simulink model "vehicle_hostmodel_2022b"  (R2022b)
settings: Solver=VariableStepAuto  StartTime=0.0  StopTime=inf  RelTol=1e-3
model workspace (MAT data in the model file):
  firstWarning = 1
  originalScenarioChecksum = '114339432DE22364D47BB28FC96DC10C'
undefined symbols (not defined in the file or in its folder): Acceleration, ActorID, AngularVelocity, curvature, DefaultGear, DEND_B, DEND_S, DEND_T, direction, DiscIntNeverNeededParam, driving, gradbp, L, LF, LR, matlabshared, MAX_BRAKE, MAX_STEER, MAX_TORQUE, MCAR, MIN_BRAKE, MIN_STEER, MIN_TORQUE, NUMD_B, NUMD_S, NUMD_T, Pitch, Position, psi_o, R, Roll, RRdamp, SceneInfo, session, sigbuilder_block, STEER_RATIO, stopSign_ID, Tdead, thetaRefs, TL_ID, TrackWidth, Ts, ts, Vdead, Velocity, WB, X_o, xRef2s, Y_o, Yaw, yRef2, yRef2s
libraries: drivingscenarioandsensors x8, slrealtimeutilitieslib x7, slrealtimeiplib x7, simulink x6, drivingvehiclecontroller x2, slpidlib x2, trackingutilitieslib x2, simulink_extras x2, robotalgslib x1, eeGeneralControl x1, mpcadaslib x1, drivinglib x1
(part 1 of 4)
settings Model: Creator=akshran  LastModifiedBy=giridhar.9
settings DataIOCC: SignalLogging=off
settings DebuggingCC: UnconnectedInputMsg=warning  UnconnectedOutputMsg=warning  UnconnectedLineMsg=warning
settings ModelReferenceCC: EnableRefExpFcnMdlSchedulingChecks=on
settings RTWCC: DLArmComputeVersion=19.05

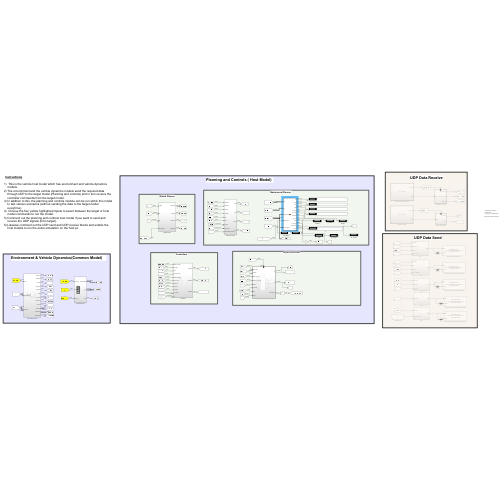
[thumbnail: Simulink's stored preview of the top-level diagram]
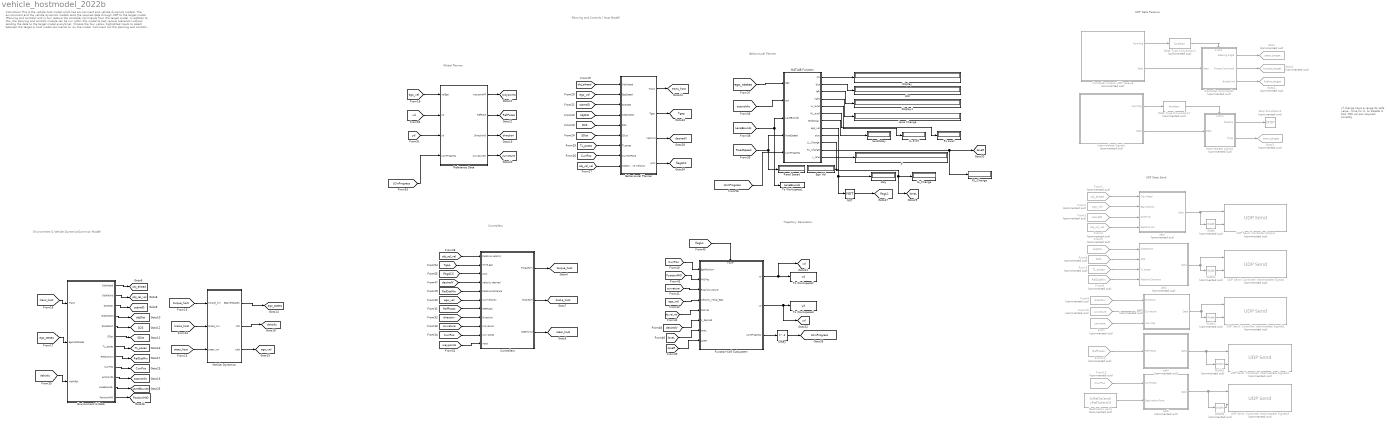
== system vehicle_hostmodel_2022b ==
  note: Global Planner
  note: xf change have a range
      | ttc safe value
      | - time for lc, to disable lc blok
      |
      | MIO vel pos required correctly
  note: Trajectory Generation
  note: Behavioural Planner
  note: Instructions
      |
      | This is the vehicle host model which has environment and vehicle dynamics models.
      | The environment and the vehicle dynamics models send the required data through UDP to the target model (Planning and controls) and in turn receive the controller commands from the target model.
      | In addition to this, the planning and controls module can be run within this model to test various scenarios (without sending the data to the target model everytime).
      | Choose the four yellow highlighted inputs to select between the target or host model commands to run the model.
      | Comment out the planning and controls host model if you want to send and receive the UDP signals (from target).
      | Likewise comment out the UDP send and UDP receive blocks and enable the host models to run the entire simulation on the host pc.
  note: Environment & Vehicle Dynamics(Common Model)
  note: UDP Data Receive
  note: UDP Data Send
  note: Planning and Controls ( Host Model)
  note: Controllers
  Behavioural Planner : Subsystem
  Controller commands : Subsystem  Commented=on
  Controller output- UDP receive : Subsystem  Commented=on
  Controllers : Subsystem
  Data Type Conversion1 : DataTypeConversion  Commented=on  OutDataTypeStr=boolean  SaturateOnIntegerOverflow=off  RndMeth=Floor
  Data Type Conversion2 : DataTypeConversion  Commented=on  OutDataTypeStr=boolean  SaturateOnIntegerOverflow=off  RndMeth=Floor
  Delay : Delay  DelayLength=1
  Destination point : Constant  Commented=on  Value=[xRef2s(end) yRef2s(end)]
  Display : Display
  Display1 : Display
  Ego Vel : Display
  Environment & Data : Subsystem
  From : From  Commented=on  GotoTag=yawrate  TagVisibility=global
  From1 : From  Commented=on  GotoTag=obj_ahead  TagVisibility=global
  From10 : From  Commented=on  GotoTag=curvature  TagVisibility=global
  From11 : From  Commented=on  GotoTag=RefPoses  TagVisibility=global
  From12 : From  Commented=on  GotoTag=CurrPos  TagVisibility=global
  From2 : From  Commented=on  GotoTag=ego_vel  TagVisibility=global
  From3 : From  Commented=on  GotoTag=sceneID  TagVisibility=global
  From4 : From  Commented=on  GotoTag=obj_rel_vel  TagVisibility=global
  From5 : From  Commented=on  GotoTag=objDist  TagVisibility=global
  From6 : From  Commented=on  GotoTag=D2S  TagVisibility=global
  From7 : From  Commented=on  GotoTag=TL_poses  TagVisibility=global
  From8 : From  Commented=on  GotoTag=RelDistMin  TagVisibility=global
  From9 : From  Commented=on  GotoTag=direction  TagVisibility=global
  Function-Call Subsystem : Subsystem  TreatAsAtomicUnit=on
  Goto : Goto  Commented=on  GotoTag=steer_target  TagVisibility=global
  Goto1 : Goto  Commented=on  GotoTag=torque_target  TagVisibility=global
  Goto2 : Goto  Commented=on  GotoTag=brake_target  TagVisibility=global
  Goto3 : Goto  Commented=on  GotoTag=trans_target  TagVisibility=global
  Intermediate Signals : Subsystem  Commented=on
  Intermediate signals : Subsystem  Commented=on
  LL avail : Display
  LL_Change : Display
  "Lane Change " : Display
  MATLAB Function : MATLAB Function  TreatAsAtomicUnit=on
  NOT : Logic  Operator=NOT  IconShape=distinctive  AllPortsSameDT=off  OutDataTypeStr=boolean
  RL avail : Display
  RL_Change : Display
  Reference Data : Subsystem  VariantControl=Stanley
  Road Speed : Display
  Stop Simulation1 : Stop  Commented=on
  To Workspace1 : ToWorkspace  VariableName=LaneBounds  SaveFormat=Timeseries  SampleTime=-1
  To Workspace2 : ToWorkspace  VariableName=xd  SampleTime=-1
      settings: Save2DSignal=2-D array (concatenate along first dimension)
  To Workspace3 : ToWorkspace  VariableName=yd  SampleTime=-1
      settings: Save2DSignal=2-D array (concatenate along first dimension)
  UDP Send: Controller Intermediate Signals : slrealtimeiplib/UDP Send  Commented=on  useHostTargetConn=on  toAddress=192.168.7.2  toPort=8002  sampleTime=0.1  enableMessage=off  ipAddress=192.168.7.2  localPort=-1
  UDP Send: Controller Intermediate Signals1 : slrealtimeiplib/UDP Send  Commented=on  useHostTargetConn=on  toAddress=192.168.7.2  toPort=8003  sampleTime=0.1  enableMessage=off  ipAddress=192.168.7.2  localPort=-1
  UDP Send: Controller Intermediate Signals2 : slrealtimeiplib/UDP Send  Commented=on  useHostTargetConn=on  toAddress=192.168.7.2  toPort=8004  sampleTime=0.1  enableMessage=off  ipAddress=192.168.7.2  localPort=-1
  UDP Send: Controller Intermediate Signals3 : slrealtimeiplib/UDP Send  Commented=on  useHostTargetConn=on  toAddress=192.168.7.2  toPort=8005  sampleTime=0.1  enableMessage=off  ipAddress=192.168.7.2  localPort=-1
  UDP Send: Controller Output : slrealtimeiplib/UDP Send  Commented=on  useHostTargetConn=on  toAddress=192.168.7.2  toPort=8001  sampleTime=0.1  enableMessage=off  ipAddress=192.168.7.2  localPort=-1
  Vehicle Dynamics : Subsystem
  Width{,1..4} (5 alike) : Width  Commented=on
  d : Display
  dist : Display
  set1 : Subsystem  Commented=on
  set2 : Subsystem  Commented=on
  set3 : Subsystem  Commented=on
  set4 : Subsystem  Commented=on
  set5 : Subsystem  Commented=on
  stay : Display
  tend2stay : Display
  tag scope: CurrPos=global, D2S=global, LCinProgress=global, LaneBounds=global, PositionMIO=global, RefPoses=global, RelDistMin=global, SDist=global, TL_poses=global, Tgap=global, VehInfo=global, actorsInfo=global, brake_host=global, curvature=global, desiredV=global, direction=global, ego_states=global, ego_vel=global, flagACC=global, flagLC=global, laneL=global, laneR=global, objDist=global, obj_ahead=global, obj_rel_vel=global, sceneID=global, steer_host=global, torque_host=global, trans_host=global, waypoints=global, xd=global, yd=global
  wires:
  Behavioural Planner/3(VelCmd) -> [desiredV]
  Width/1 -> UDP Send: Controller Output/2
  Width1/1 -> UDP Send: Controller Intermediate Signals/2
  set1/1(Data) -> Width/1, UDP Send: Controller Output/1
  set2/1(Data) -> UDP Send: Controller Intermediate Signals/1, Width1/1
  set3/1(Data) -> UDP Send: Controller Intermediate Signals1/1, Width2/1
  Width2/1 -> UDP Send: Controller Intermediate Signals1/2
  Width3/1 -> UDP Send: Controller Intermediate Signals2/2
  set4/1(Data) -> Width3/1, UDP Send: Controller Intermediate Signals2/1
  set5/1(Data) -> Width4/1, UDP Send: Controller Intermediate Signals3/1
  Width4/1 -> UDP Send: Controller Intermediate Signals3/2
  From/1 -> set3/3(yaw rate)
  Controller output- UDP receive/2(Data) -> Controller commands/1(Data)
  Controller output- UDP receive/1(NumMsg) -> Data Type Conversion2/1
  Data Type Conversion2/1 -> Controller commands/Enable
  Data Type Conversion1/1 -> Intermediate signals/Enable
  Intermediate Signals/1(NumMsg) -> Data Type Conversion1/1
  Intermediate Signals/2(Data) -> Intermediate signals/1(Data)
  Intermediate signals/1(StopSim) -> Stop Simulation1/1
  Destination point/1 -> set5/2(Destination Point)
  Controller commands/1(Steering Angle) -> Goto/1
  Controller commands/2(Torque Command) -> Goto1/1
  Controller commands/3(BrakeCmd) -> Goto2/1
  Intermediate signals/2(Trans) -> Goto3/1
  Controllers/1(TorgueCm) -> [torque_host]
  Controllers/2(BrakeCm) -> [brake_host]
  Controllers/3(SteerCmd) -> [steer_host]
  Environment & Data/1(ObjAhead) -> [obj_ahead]
  Environment & Data/2(ObjRelVel) -> [obj_rel_vel]
  Environment & Data/3(SceneID) -> [sceneID]
  Environment & Data/4(ObjectDist) -> [objDist]
  Environment & Data/6(SDist) -> [SDist]
  Environment & Data/5(SceneDist) -> [D2S]
  Environment & Data/7(TL_poses) -> [TL_poses]
  Vehicle Dynamics/1(EgoVehStates) -> [ego_states]
  Vehicle Dynamics/3(xdot) -> [ego_vel]
  Environment & Data/8(RelDistmin) -> [RelDistMin]
  Vehicle Dynamics/2(Info) -> [VehInfo]
  Behavioural Planner/1(Trans) -> [trans_host]
  From1/1 -> set1/1(Obj Ahead)
  From2/1 -> set1/2(Ego Velocity)
  From3/1 -> set1/3(Scene ID)
  From4/1 -> set1/4(Relative Vel)
  From5/1 -> set2/1(ObjectDist)
  From6/1 -> set2/2(D2S)
  From7/1 -> set2/3(TL poses)
  From8/1 -> set2/4(Relative Distance)
  From9/1 -> set3/1(Direction)
  From10/1 -> set3/2(Curvature)
  From11/1 -> set4/1(Ref Poses)
  From12/1 -> set5/1(CurrPoses)
  [torque_host] -> Vehicle Dynamics/1(torque_cm)
  [brake_host] -> Vehicle Dynamics/2(brake_cm)
  [steer_host] -> Vehicle Dynamics/3(steer_cm)
  [trans_host] -> Environment & Data/1(Trans)
  [ego_states] -> Environment & Data/2(EgoVehStates)
  [obj_ahead] -> Behavioural Planner/1(ObjAhead)
  [ego_vel] -> Behavioural Planner/2(EgoSpeed)
  [sceneID] -> Behavioural Planner/3(SceneID)
  [objDist] -> Behavioural Planner/4(ObjectDist)
  [D2S] -> Behavioural Planner/5(D2S)
  [SDist] -> Behavioural Planner/6(SDist)
  [TL_poses] -> Behavioural Planner/7(TLposes)
  [CurrPos] -> Behavioural Planner/8(CurrentPose)
  [obj_rel_vel] -> Behavioural Planner/9(Object Relative Velocity)
  [obj_rel_vel] -> Controllers/1(Relative velocity)
  [RelDistMin] -> Controllers/5(Relative distance)
  [ego_vel] -> Controllers/6(CurrVelocity)
  [RefPoses] -> Controllers/7(RefPoses)
  [direction] -> Controllers/8(Direction)
  [curvature] -> Controllers/9(Curvature)
  [CurrPos] -> Controllers/10(curr poses)
  [VehInfo] -> Environment & Data/3(VehFdbk)
  Environment & Data/9(CurrPos) -> [CurrPos]
  Environment & Data/10(actorsinfo) -> [actorsInfo]
  [ego_states] -> MATLAB Function/1(ego)
  [actorsInfo] -> MATLAB Function/2(act)
  MATLAB Function/1(ttc) -> Display/1
  Environment & Data/11(LaneBounds) -> [LaneBounds]
  [LaneBounds] -> MATLAB Function/3(LaneBounds), To Workspace1/1
  MATLAB Function/3(left) -> Display1/1
  MATLAB Function/4(right) -> "Lane Change "/1
  MATLAB Function/2(dist) -> dist/1
  [RoadSpeed] -> Road Speed/1, MATLAB Function/4(RoadSpeed)
  MATLAB Function/8(ego_vel) -> Ego Vel/1
  MATLAB Function/6(RL_avail) -> RL avail/1
  MATLAB Function/5(LL_avail) -> LL avail/1
  MATLAB Function/7(tend2stay) -> tend2stay/1
  MATLAB Function/9(stay) -> NOT/1, stay/1
  MATLAB Function/10(LL_Change) -> LL_Change/1, [laneL]
  MATLAB Function/11(RL_Change) -> RL_Change/1, [laneR]
  MATLAB Function/12(y_lane) -> d/1
  [CurrPos] -> Function-Call Subsystem/1(EgoPosition)
  [curvature] -> Function-Call Subsystem/3(Road Curvature)
  [ego_vel] -> Function-Call Subsystem/4(Velocity_Initial_Ego)
  Environment & Data/12(PositionMIO) -> [PositionMIO]
  [PositionMIO] -> Function-Call Subsystem/2(MIOPos)
  [obj_rel_vel] -> Function-Call Subsystem/5(MIOVel)
  NOT/1 -> [flagLC]
  Function-Call Subsystem/1(xd) -> [xd], To Workspace2/1
  Function-Call Subsystem/2(yd) -> [yd], To Workspace3/1
  [desiredV] -> Function-Call Subsystem/6(V_desired)
  [desiredV] -> Controllers/4(velocity desired)
  [laneR] -> Function-Call Subsystem/8(laneR)
  [laneL] -> Function-Call Subsystem/7(laneL)
  [flagLC] -> Function-Call Subsystem/Trigger
  [ego_vel] -> Reference Data/1(velEgo)
  Reference Data/1(waypointPP) -> [waypoints]
  Reference Data/2(RefPose) -> [RefPoses]
  Reference Data/3(DirectionO) -> [direction]
  [xd] -> Reference Data/2(xd)
  [yd] -> Reference Data/3(yd)
  [waypoints] -> Controllers/11(Input)
  Reference Data/4(CurvatureO) -> [curvature]
  [LCinProgress] -> Reference Data/4(LCinProgress)
  Behavioural Planner/2(Tgap) -> [Tgap]
  Behavioural Planner/4(ACC) -> [flagACC]
  [Tgap] -> Controllers/2(Time gap)
  [flagACC] -> Controllers/3(ACC)
  Function-Call Subsystem/3(LCinProgress) -> Delay/1
  Delay/1 -> [LCinProgress]
  [LCinProgress] -> MATLAB Function/5(LCinProgress)

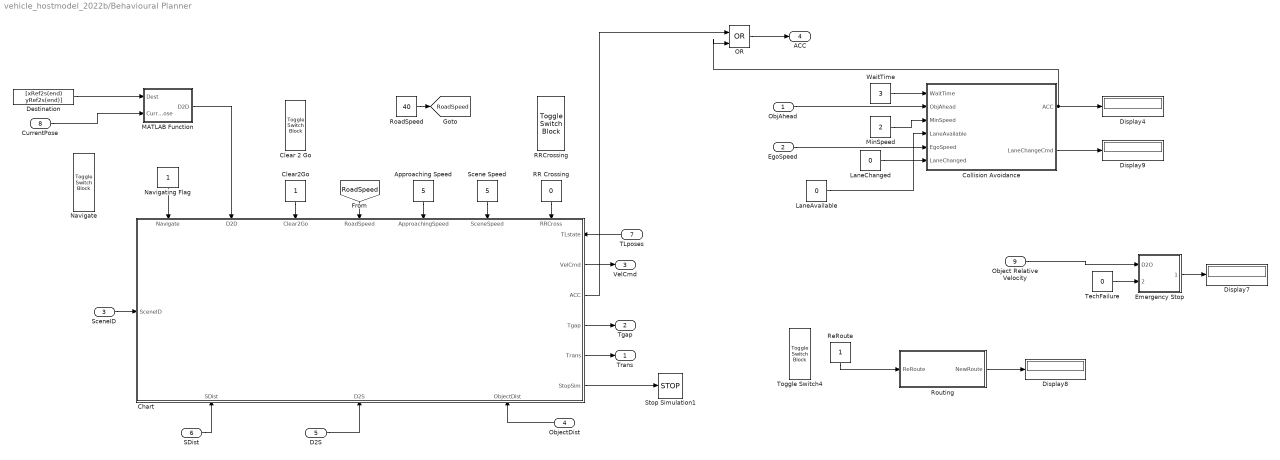
== system vehicle_hostmodel_2022b/Behavioural Planner ==
  ObjAhead : Inport
  EgoSpeed : Inport  Port=2
  SceneID : Inport  Port=3
  ObjectDist : Inport  Port=4
  D2S : Inport  Port=5
  SDist : Inport  Port=6
  TLposes : Inport  Port=7
  CurrentPose : Inport  Port=8
  Object Relative Velocity : Inport  Port=9
  Approaching Speed : Constant  Value=5
  Chart : Stateflow chart  TreatAsAtomicUnit=on
      settings: PortSchema="{\"entries\":[{\"content\":{\"sides\":[{\"content\":{\"connectorIds\":[\"In12\"]},\"type\":\"ConnectorPlacement.EquallySpacedRectSide\",\"uuid\":\"81aca70f-0947-49fb-b60a-be241e44193b\"},{\"content\":{\"connectorIds\":[\"In1\",\"Out1\",\"Out2\",\"Out3\",\"Out4\",\"Out5\"],\"side\":\"RIGHT\"},\"type\":\"ConnectorPlacement.EquallySpacedRectSide\",\"uuid\":\"e7b9645e-3711-4964-ac9b-0199dd335e99\"},{\"content\":{\"connectorIds\":[\"In8\",\"In9\",\"In10\",\"In11\",\"In2\",\"In4\",\"In6\"],\"side\":\"TOP\"},\"type\":\"ConnectorPlacement.EquallySpacedRectSide\",\"uuid\":\"6876f024-944b-4540-9404-d68f37763657\"},{\"content\":{\"connectorIds\":[\"In5\",\"In7\",\"In3\"],\"side\":\"BOTTOM\"},\"type\":\"ConnectorPlacement.EquallySpacedRectSide\",\"uuid\":\"44acab73-cdde-4edf-95df-27422644ccab\"}]},\"type\":\"ConnectorPlacement.EquallySpacedConnector\",\"uuid\":\"d2c31c01-e447-43db-8d2b-8b98a0ca291a\"}],\"packageUris\":[\"http://schema.mathworks.com/mf0/Connector/R2020b\"],\"version\":\"1.0\"}"
  Clear 2 Go : ToggleSwitchBlock
      settings: Values={{'Off', 'On'}, [0 1]}
  Clear2Go : Constant
  Collision Avoidance : Stateflow chart  TreatAsAtomicUnit=on
  Destination : Constant  Value=[xRef2s(end) yRef2s(end)]
  Display{4,7..9} (4 alike) : Display
  Emergency Stop : Stateflow chart  TreatAsAtomicUnit=on
  LaneAvailable : Constant  Value=0
  LaneChanged : Constant  Value=0
  MATLAB Function : MATLAB Function  TreatAsAtomicUnit=on
  MinSpeed : Constant  Value=2
  Navigate : ToggleSwitchBlock
      settings: Values={{'Off', 'On'}, [0 1]}
  Navigating Flag : Constant
  OR : Logic  Operator=OR  IconShape=distinctive  AllPortsSameDT=off  OutDataTypeStr=fixdt(1,16)
  RR Crossing : Constant  Value=0
  RRCrossing : ToggleSwitchBlock
      settings: Values={{'Off', 'On'}, [0 1]}
  ReRoute : Constant
  RoadSpeed : Constant  Value=40
  Routing : Stateflow chart  TreatAsAtomicUnit=on
  Scene Speed : Constant  Value=5
  Stop Simulation1 : Stop
  TechFailure : Constant  Value=0
  Toggle Switch4 : ToggleSwitchBlock
      settings: Values={{'Off', 'On'}, [0 1]}
  WaitTime : Constant  Value=3
  Trans : Outport
  Tgap : Outport  Port=2
  VelCmd : Outport  Port=3
  ACC : Outport  Port=4
  tag scope: RoadSpeed=global
  wires:
  Clear2Go/1 -> Chart/10(Clear2Go)
  Routing/1(NewRoute) -> Display8/1
  ObjectDist/1 -> Chart/3(ObjectDist)
  WaitTime/1 -> Collision Avoidance/1(WaitTime)
  Navigating Flag/1 -> Chart/8(Navigate)
  Approaching Speed/1 -> Chart/2(ApproachingSpeed)
  Scene Speed/1 -> Chart/4(SceneSpeed)
  EgoSpeed/1 -> Collision Avoidance/5(EgoSpeed)
  ReRoute/1 -> Routing/1(ReRoute)
  Collision Avoidance/2(LaneChangeCmd) -> Display9/1
  LaneAvailable/1 -> Collision Avoidance/4(LaneAvailable)
  CurrentPose/1 -> MATLAB Function/2(CurrentPose)
  RR Crossing/1 -> Chart/6(RRCross)
  MinSpeed/1 -> Collision Avoidance/3(MinSpeed)
  LaneChanged/1 -> Collision Avoidance/6(LaneChanged)
  [RoadSpeed] -> Chart/11(RoadSpeed)
  ObjAhead/1 -> Collision Avoidance/2(ObjAhead)
  Destination/1 -> MATLAB Function/1(Dest)
  SceneID/1 -> Chart/12(SceneID)
  MATLAB Function/1(D2D) -> Chart/9(D2D)
  Chart/5(StopSim) -> Stop Simulation1/1
  Chart/4(Trans) -> Trans/1
  TLposes/1 -> Chart/1(TLstate)
  Chart/1(VelCmd) -> VelCmd/1
  SDist/1 -> Chart/5(SDist)
  D2S/1 -> Chart/7(D2S)
  Chart/3(Tgap) -> Tgap/1
  TechFailure/1 -> Emergency Stop/2(TechFailure)
  Emergency Stop/1(EStop) -> Display7/1
  Object Relative Velocity/1 -> Emergency Stop/1(D2O)
  Collision Avoidance/1(ACC) -> OR/2, Display4/1
  OR/1 -> ACC/1
  Chart/2(ACC) -> OR/1
  RoadSpeed/1 -> [RoadSpeed]

== system vehicle_hostmodel_2022b/Controller commands ==
  Data : Inport
  Enable : EnablePort
  "Byte Unpacking " : slrealtimeutilitieslib/Byte Unpacking  MaskUnpackedDataTypes={'double', 'double', 'double'}  MaskUnpackedDataSizes={[1], [1], [1]}  MaskAlignment=1
  Steering Angle : Outport
  Torque Command : Outport  Port=2
  BrakeCmd : Outport  Port=3
  wires:
  Data/1 -> "Byte Unpacking "/1
  "Byte Unpacking "/1 -> Steering Angle/1  "Steering angle"
  "Byte Unpacking "/2 -> Torque Command/1  "Longitudinal velocity"
  "Byte Unpacking "/3 -> BrakeCmd/1  "BrakeCmd"

== system vehicle_hostmodel_2022b/Controller output- UDP receive ==
  Compare To Constant : simulink/Logic and Bit Operations/Compare To Constant  relop===  const=24  OutDataTypeStr=boolean
  Constant : Constant
  Subtract : Sum  Inputs=+-
  UDP Receive2 : slrealtimeiplib/UDP Receive  useHostTargetConn=on  ipAddress=192.168.7.2  localPort=8016  rcvWidth=24  rcvFmAny=off  fmAddress=192.168.7.2  sampleTime=-1  enableMessage=off  maxPackets=1
  While Iterator : WhileIterator  WhileBlockType=do-while  ResetStates=reset  ShowIterationPort=on
  NumMsg : Outport
  Data : Outport  Port=2
  wires:
  Compare To Constant/1 -> While Iterator/1
  UDP Receive2/1 -> Data/1
  Constant/1 -> Subtract/2
  Subtract/1 -> NumMsg/1
  UDP Receive2/2 -> Compare To Constant/1
  While Iterator/1 -> Subtract/1

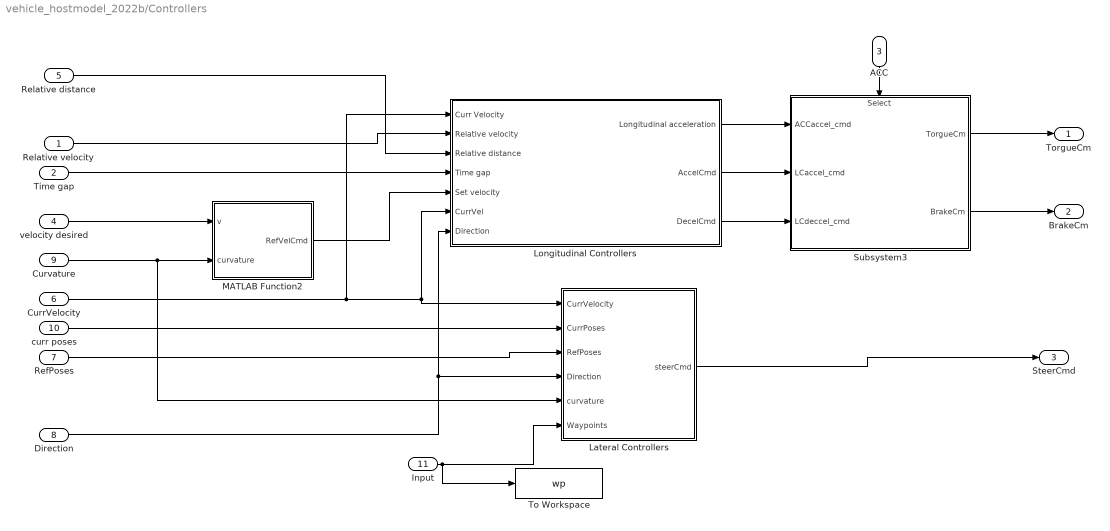
== system vehicle_hostmodel_2022b/Controllers ==
  Relative velocity : Inport
  Time gap : Inport  Port=2
  ACC : Inport  Port=3
  velocity desired : Inport  Port=4
  Relative distance : Inport  Port=5
  CurrVelocity : Inport  Port=6
  RefPoses : Inport  Port=7
  Direction : Inport  Port=8
  Curvature : Inport  Port=9
  curr poses : Inport  Port=10
  Input : Inport  Port=11
  Lateral Controllers : Subsystem
  Longitudinal Controllers : Subsystem
  MATLAB Function2 : MATLAB Function  TreatAsAtomicUnit=on
  Subsystem3 : Subsystem
      settings: PortSchema="{\"entries\":[{\"content\":{\"sides\":[{\"content\":{\"connectorIds\":[\"In1\",\"In2\",\"In3\"]},\"type\":\"ConnectorPlacement.EquallySpacedRectSide\",\"uuid\":\"a23b1a10-3bcb-40a0-900c-c9a3f160b173\"},{\"content\":{\"connectorIds\":[\"Out1\",\"Out2\"],\"side\":\"RIGHT\"},\"type\":\"ConnectorPlacement.EquallySpacedRectSide\",\"uuid\":\"88840b66-912f-4184-aeec-297642319416\"},{\"content\":{\"connectorIds\":[\"In4\"],\"side\":\"TOP\"},\"type\":\"ConnectorPlacement.EquallySpacedRectSide\",\"uuid\":\"37a03ca9-b065-473e-b290-3b07703c6005\"}]},\"type\":\"ConnectorPlacement.EquallySpacedConnector\",\"uuid\":\"5bfc7c71-8f7a-4cba-a168-7eeca22a2fcb\"}],\"packageUris\":[\"http://schema.mathworks.com/mf0/Connector/R2020b\"],\"version\":\"1.0\"}"
  To Workspace : ToWorkspace  VariableName=wp  SampleTime=-1
  TorgueCm : Outport
  BrakeCm : Outport  Port=2
  SteerCmd : Outport  Port=3
  wires:
  Longitudinal Controllers/1(Longitudinal acceleration) -> Subsystem3/1(ACCaccel_cmd)
  Curvature/1 -> MATLAB Function2/2(curvature), Lateral Controllers/5(curvature)
  Relative velocity/1 -> Longitudinal Controllers/2(Relative velocity)
  MATLAB Function2/1(RefVelCmd) -> Longitudinal Controllers/5(Set velocity)
  Direction/1 -> Longitudinal Controllers/7(Direction), Lateral Controllers/4(Direction)
  RefPoses/1 -> Lateral Controllers/3(RefPoses)
  velocity desired/1 -> MATLAB Function2/1(v)
  Longitudinal Controllers/2(AccelCmd) -> Subsystem3/2(LCaccel_cmd)
  Longitudinal Controllers/3(DecelCmd) -> Subsystem3/3(LCdeccel_cmd)
  CurrVelocity/1 -> Longitudinal Controllers/1(Curr Velocity), Longitudinal Controllers/6(CurrVel), Lateral Controllers/1(CurrVelocity)
  Time gap/1 -> Longitudinal Controllers/4(Time gap)
  Relative distance/1 -> Longitudinal Controllers/3(Relative distance)
  Lateral Controllers/1(steerCmd) -> SteerCmd/1
  ACC/1 -> Subsystem3/4(Select)
  curr poses/1 -> Lateral Controllers/2(CurrPoses)
  Subsystem3/1(TorgueCm) -> TorgueCm/1
  Subsystem3/2(BrakeCm) -> BrakeCm/1
  Input/1 -> To Workspace/1, Lateral Controllers/6(Waypoints)

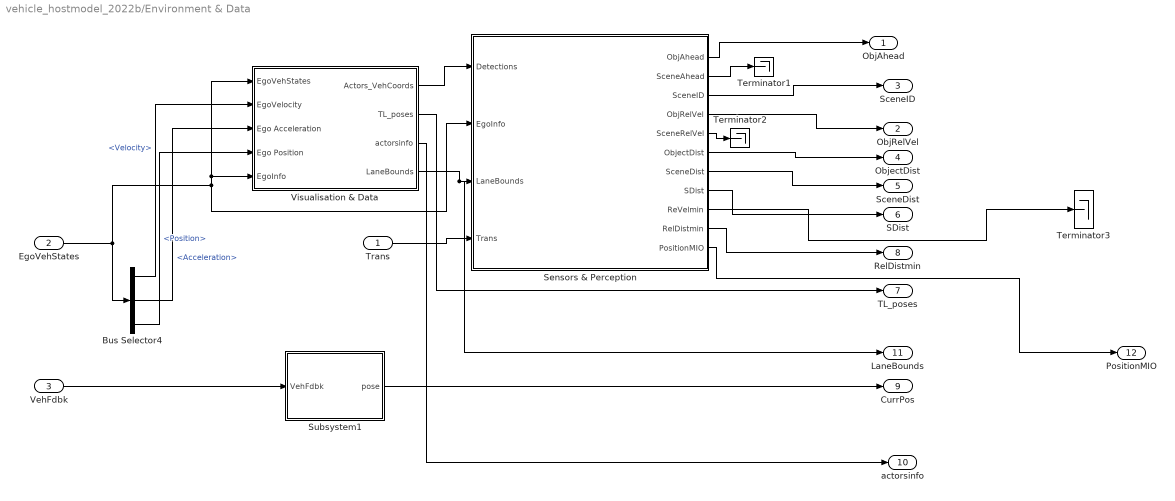
== system vehicle_hostmodel_2022b/Environment & Data ==
  Trans : Inport
  EgoVehStates : Inport  Port=2
  VehFdbk : Inport  Port=3
  Bus Selector4 : BusSelector  OutputSignals=Velocity,Acceleration,Position
  Sensors & Perception : Subsystem
  Subsystem1 : Subsystem
  Terminator1 : Terminator
  Terminator2 : Terminator
  Terminator3 : Terminator
  Visualisation & Data : Subsystem
  ObjAhead : Outport
  ObjRelVel : Outport  Port=2
  SceneID : Outport  Port=3
  ObjectDist : Outport  Port=4
  SceneDist : Outport  Port=5
  SDist : Outport  Port=6
  TL_poses : Outport  Port=7
  RelDistmin : Outport  Port=8
  CurrPos : Outport  Port=9
  actorsinfo : Outport  Port=10
  LaneBounds : Outport  Port=11
  PositionMIO : Outport  Port=12
  wires:
  Bus Selector4/3 -> Visualisation & Data/4(Ego Position)  "<Position>"
  Sensors & Perception/1(ObjAhead) -> ObjAhead/1
  Bus Selector4/1 -> Visualisation & Data/2(EgoVelocity)  "<Velocity>"
  Visualisation & Data/1(Actors_VehCoords) -> Sensors & Perception/1(Detections)
  Sensors & Perception/5(SceneRelVel) -> Terminator2/1
  Sensors & Perception/2(SceneAhead) -> Terminator1/1
  Sensors & Perception/6(ObjectDist) -> ObjectDist/1
  Bus Selector4/2 -> Visualisation & Data/3(Ego Acceleration)  "<Acceleration>"
  Sensors & Perception/9(ReVelmin) -> Terminator3/1
  EgoVehStates/1 -> Visualisation & Data/5(EgoInfo), Visualisation & Data/1(EgoVehStates), Sensors & Perception/2(EgoInfo), Bus Selector4/1
  Sensors & Perception/4(ObjRelVel) -> ObjRelVel/1
  Visualisation & Data/2(TL_poses) -> TL_poses/1
  Sensors & Perception/3(SceneID) -> SceneID/1
  Sensors & Perception/8(SDist) -> SDist/1
  Sensors & Perception/7(SceneDist) -> SceneDist/1
  Trans/1 -> Sensors & Perception/4(Trans)
  Sensors & Perception/10(RelDistmin) -> RelDistmin/1
  VehFdbk/1 -> Subsystem1/1(VehFdbk)
  Subsystem1/1(pose) -> CurrPos/1
  Visualisation & Data/3(actorsinfo) -> actorsinfo/1
  Visualisation & Data/4(LaneBounds) -> LaneBounds/1, Sensors & Perception/3(LaneBounds)
  Sensors & Perception/11(PositionMIO) -> PositionMIO/1

== system vehicle_hostmodel_2022b/Function-Call Subsystem ==
  EgoPosition : Inport
  MIOPos : Inport  Port=2
  Road Curvature : Inport  Port=3
  Velocity_Initial_Ego : Inport  Port=4
  MIOVel : Inport  Port=5
  V_desired : Inport  Port=6
  laneL : Inport  Port=7
  laneR : Inport  Port=8
  function : TriggerPort  VariantControl=(inherit)  ShowOutputPort=on
  MATLAB Function : MATLAB Function  TreatAsAtomicUnit=on
  Scope : Scope  NumInputPorts=2
  xd : Outport
  yd : Outport  Port=2
  LCinProgress : Outport  Port=3  InitialOutput=0
  wires:
  EgoPosition/1 -> MATLAB Function/1(EgoPosition)
  MIOPos/1 -> MATLAB Function/2(MIOPos)
  Road Curvature/1 -> MATLAB Function/3(curvature)
  MIOVel/1 -> MATLAB Function/4(MIOVel)
  Velocity_Initial_Ego/1 -> MATLAB Function/5(V_i)
  MATLAB Function/1(xd) -> Scope/1, xd/1
  MATLAB Function/2(yd) -> yd/1, Scope/2
  V_desired/1 -> MATLAB Function/8(V_desired)
  laneL/1 -> MATLAB Function/6(laneL)
  laneR/1 -> MATLAB Function/7(laneR)
  MATLAB Function/3(LCinProgress) -> LCinProgress/1

== system vehicle_hostmodel_2022b/Intermediate Signals ==
  Compare To Constant : simulink/Logic and Bit Operations/Compare To Constant  relop===  const=16  OutDataTypeStr=boolean
  Constant : Constant
  Subtract : Sum  Inputs=+-
  UDP Receive2 : slrealtimeiplib/UDP Receive  useHostTargetConn=on  ipAddress=192.168.7.2  localPort=8017  rcvWidth=16  rcvFmAny=off  fmAddress=192.168.7.2  sampleTime=-1  enableMessage=off  maxPackets=1
  While Iterator : WhileIterator  WhileBlockType=do-while  ResetStates=reset  ShowIterationPort=on
  NumMsg : Outport
  Data : Outport  Port=2
  wires:
  While Iterator/1 -> Subtract/1
  UDP Receive2/2 -> Compare To Constant/1
  Subtract/1 -> NumMsg/1
  Constant/1 -> Subtract/2
  UDP Receive2/1 -> Data/1
  Compare To Constant/1 -> While Iterator/1

== system vehicle_hostmodel_2022b/Intermediate signals ==
  Data : Inport
  Enable : EnablePort
  "Byte Unpacking " : slrealtimeutilitieslib/Byte Unpacking  MaskUnpackedDataTypes={'double', 'double'}  MaskUnpackedDataSizes={[1], [1]}  MaskAlignment=1
  StopSim : Outport
  Trans : Outport  Port=2
  wires:
  "Byte Unpacking "/2 -> Trans/1  "Trans"
  "Byte Unpacking "/1 -> StopSim/1  "StopSim"
  Data/1 -> "Byte Unpacking "/1

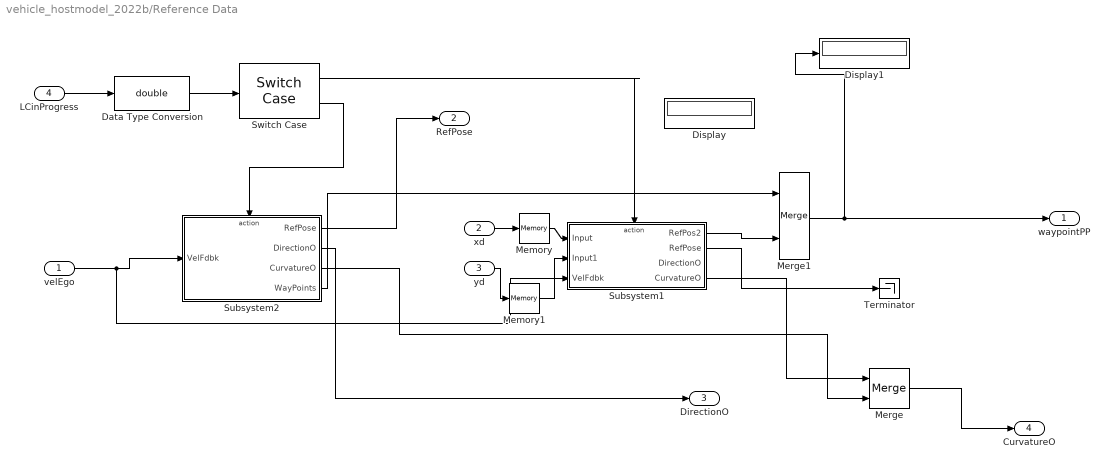
== system vehicle_hostmodel_2022b/Reference Data ==
  velEgo : Inport
  xd : Inport  Port=2
  yd : Inport  Port=3
  LCinProgress : Inport  Port=4
  Data Type Conversion : DataTypeConversion  OutDataTypeStr=double  RndMeth=Round  SaturateOnIntegerOverflow=off
  Display : Display
  Display1 : Display
  Memory : Memory  InheritSampleTime=on
  Memory1 : Memory  InheritSampleTime=on
  Merge : Merge
  Merge1 : Merge
  Subsystem1 : Subsystem
  Subsystem2 : Subsystem
  Switch Case : SwitchCase  CaseConditions={1,0}  ShowDefaultCase=off
  Terminator : Terminator
  waypointPP : Outport
  RefPose : Outport  Port=2
  DirectionO : Outport  Port=3
  CurvatureO : Outport  Port=4
  wires:
  velEgo/1 -> Subsystem1/3(VelFdbk), Subsystem2/1(VelFdbk)
  Subsystem2/4(WayPoints) -> Merge1/1
  Subsystem1/1(RefPos2) -> Merge1/2
  Merge1/1 -> Display1/1, waypointPP/1
  Subsystem2/1(RefPose) -> RefPose/1
  Subsystem2/2(DirectionO) -> DirectionO/1
  Switch Case/2 -> Subsystem2/Action
  Switch Case/1 -> Subsystem1/Action
  Subsystem1/4(CurvatureO) -> Merge/1
  Merge/1 -> CurvatureO/1
  Subsystem2/3(CurvatureO) -> Merge/2
  Memory/1 -> Subsystem1/1(Input)
  xd/1 -> Memory/1
  Memory1/1 -> Subsystem1/2(Input1)
  yd/1 -> Memory1/1
  Data Type Conversion/1 -> Switch Case/1
  Subsystem1/2(RefPose) -> Terminator/1
  LCinProgress/1 -> Data Type Conversion/1

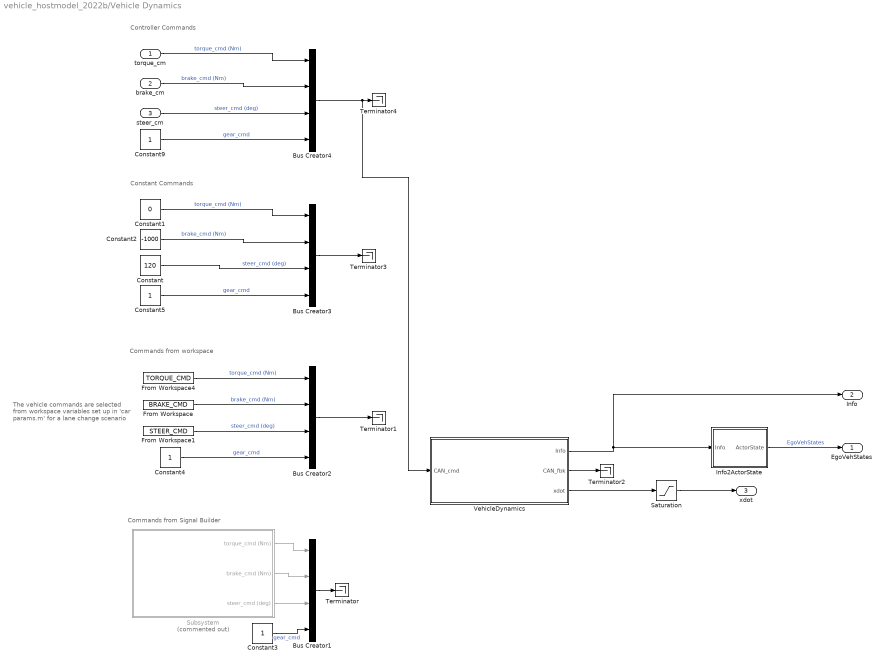
== system vehicle_hostmodel_2022b/Vehicle Dynamics ==
  note: Constant Commands
  note: Commands from workspace
  note: Commands from Signal Builder
  note: The vehicle commands are selected from workspace variables set up in 'car params.m' for a lane change scenario
  note: Controller Commands
  torque_cm : Inport
  brake_cm : Inport  Port=2
  steer_cm : Inport  Port=3
  Bus Creator{1..4} (4 alike) : BusCreator  Inputs=4
  Constant : Constant  Value=120
  Constant1 : Constant  Value=0
  Constant2 : Constant  Value=-1000
  Constant{3..5,9} (4 alike) : Constant
  From Workspace : FromWorkspace  VariableName=BRAKE_CMD  SampleTime=ts
  From Workspace1 : FromWorkspace  VariableName=STEER_CMD  SampleTime=ts
  From Workspace4 : FromWorkspace  VariableName=TORQUE_CMD  SampleTime=ts
  Info2ActorState : Subsystem
  Saturation : Saturate  UpperLimit=inf  LowerLimit=0.001
  Subsystem : Subsystem  Commented=on
  Terminator{,1..4} (5 alike) : Terminator
  VehicleDynamics : Subsystem  mask{InitPosition=[X_o Y_o 0], InitSpeed=0, InitYaw=psi_o}
      mask prompts: InitPosition "Initial Position (m)"; InitSpeed "Initial Speed (m/s)"; InitYaw "Init Yaw (rad)"
  EgoVehStates : Outport
  Info : Outport  Port=2
  xdot : Outport  Port=3
  wires:
  Bus Creator2/1 -> Terminator1/1
  VehicleDynamics/2(CAN_fbk) -> Terminator2/1
  VehicleDynamics/1(Info) -> Info/1, Info2ActorState/1(Info)
  Constant/1 -> Bus Creator3/3  "steer_cmd (deg)"
  Info2ActorState/1(ActorState) -> EgoVehStates/1  "EgoVehStates"
  Constant1/1 -> Bus Creator3/1  "torque_cmd (Nm)"
  Constant2/1 -> Bus Creator3/2  "brake_cmd (Nm)"
  VehicleDynamics/3(xdot) -> Saturation/1
  Subsystem/1(torque_cmd (Nm)) -> Bus Creator1/1
  Subsystem/2(brake_cmd (Nm)) -> Bus Creator1/2
  Subsystem/3(steer_cmd (deg)) -> Bus Creator1/3
  Constant3/1 -> Bus Creator1/4  "gear_cmd"
  Constant4/1 -> Bus Creator2/4  "gear_cmd"
  From Workspace/1 -> Bus Creator2/2  "brake_cmd (Nm)"
  From Workspace1/1 -> Bus Creator2/3  "steer_cmd (deg)"
  From Workspace4/1 -> Bus Creator2/1  "torque_cmd (Nm)"
  Constant5/1 -> Bus Creator3/4  "gear_cmd"
  Bus Creator1/1 -> Terminator/1
  brake_cm/1 -> Bus Creator4/2  "brake_cmd (Nm)"
  Constant9/1 -> Bus Creator4/4  "gear_cmd"
  torque_cm/1 -> Bus Creator4/1  "torque_cmd (Nm)"
  steer_cm/1 -> Bus Creator4/3  "steer_cmd (deg)"
  Bus Creator3/1 -> Terminator3/1
  Bus Creator4/1 -> VehicleDynamics/1(CAN_cmd), Terminator4/1
  Saturation/1 -> xdot/1

== system vehicle_hostmodel_2022b/set1 ==
  Obj Ahead : Inport
  Ego Velocity : Inport  Port=2
  Scene ID : Inport  Port=3
  Relative Vel : Inport  Port=4
  Byte Packing : slrealtimeutilitieslib/Byte Packing  MaskPackedDataType=uint8  MaskUnpackedDataTypes={'double', 'double','double','double'}  MaskAlignment=1
  Data : Outport
  wires:
  Ego Velocity/1 -> Byte Packing/2
  Byte Packing/1 -> Data/1
  Obj Ahead/1 -> Byte Packing/1
  Scene ID/1 -> Byte Packing/3
  Relative Vel/1 -> Byte Packing/4

== system vehicle_hostmodel_2022b/set2 ==
  ObjectDist : Inport
  D2S : Inport  Port=2
  TL poses : Inport  Port=3
  Relative Distance : Inport  Port=4
  Byte Packing1 : slrealtimeutilitieslib/Byte Packing  MaskPackedDataType=uint8  MaskUnpackedDataTypes={'double', 'double','double','double'}  MaskAlignment=1
  Data : Outport
  wires:
  Byte Packing1/1 -> Data/1
  ObjectDist/1 -> Byte Packing1/1
  D2S/1 -> Byte Packing1/2
  TL poses/1 -> Byte Packing1/4
  Relative Distance/1 -> Byte Packing1/3

== system vehicle_hostmodel_2022b/set3 ==
  Direction : Inport
  Curvature : Inport  Port=2
  yaw rate : Inport  Port=3
  Byte Packing1 : slrealtimeutilitieslib/Byte Packing  MaskPackedDataType=uint8  MaskUnpackedDataTypes={'double', 'double', 'double'}  MaskAlignment=1
  Data : Outport
  wires:
  Curvature/1 -> Byte Packing1/2
  Direction/1 -> Byte Packing1/1
  Byte Packing1/1 -> Data/1
  yaw rate/1 -> Byte Packing1/3

== system vehicle_hostmodel_2022b/set4 ==
  Ref Poses : Inport
  Byte Packing1 : slrealtimeutilitieslib/Byte Packing  MaskPackedDataType=uint8  MaskUnpackedDataTypes={'double'}  MaskAlignment=1
  Data : Outport
  wires:
  Byte Packing1/1 -> Data/1
  Ref Poses/1 -> Byte Packing1/1

== system vehicle_hostmodel_2022b/set5 ==
  CurrPoses : Inport
  Destination Point : Inport  Port=2
  Byte Packing1 : slrealtimeutilitieslib/Byte Packing  MaskPackedDataType=uint8  MaskUnpackedDataTypes={'double','double'}  MaskAlignment=1
  Data : Outport
  wires:
  CurrPoses/1 -> Byte Packing1/1
  Byte Packing1/1 -> Data/1
  Destination Point/1 -> Byte Packing1/2

== system vehicle_hostmodel_2022b/Controllers/Lateral Controllers ==
  note: include toggle logic
  CurrVelocity : Inport
  CurrPoses : Inport  Port=2
  RefPoses : Inport  Port=3
  Direction : Inport  Port=4
  curvature : Inport  Port=5
  Waypoints : Inport  Port=6
  Constant5 : Constant  Value=0
  Gain1 : Gain  Gain=180/pi
  Gain2 : Gain  Gain=1/STEER_RATIO
  Lateral Controller Stanley : drivingvehiclecontroller/Lateral Controller Stanley  ModelType=Dynamic bicycle model  PositionGainF=2.5  PositionGainR=2.5  YawRateGain=0.2  DelayGain=0.2  VehicleMass=MCAR  Lf=LF  Lr=LR  TireStiffness=5e3  Wheelbase=3  MaxSteeringAngle=80
  Pure Pursuit Controller1 : Subsystem
  Subsystem1 : Subsystem
  Switch : Switch  Criteria=u2 > Threshold  SaturateOnIntegerOverflow=off  InputSameDT=off
  Toggle Switch1 : ToggleSwitchBlock
      settings: Values={{'Off', 'On'}, [0 1]}
  Unit Delay : UnitDelay  SampleTime=-1  HasFrameUpgradeWarning=on
  steerCmd : Outport
  wires:
  Direction/1 -> Lateral Controller Stanley/4
  [yawrate] -> Gain1/1
  CurrPoses/1 -> Pure Pursuit Controller1/1(currentPose), Subsystem1/1(pose), Lateral Controller Stanley/2
  Gain1/1 -> Lateral Controller Stanley/6
  CurrVelocity/1 -> Subsystem1/2(velocity), Lateral Controller Stanley/3
  RefPoses/1 -> Lateral Controller Stanley/1
  Switch/1 -> Gain2/1
  Lateral Controller Stanley/1 -> Switch/1, Unit Delay/1
  Constant5/1 -> Switch/2
  Gain2/1 -> steerCmd/1
  Waypoints/1 -> Subsystem1/3(Input), Pure Pursuit Controller1/2(Waypoints)
  Subsystem1/1(steerCmd) -> Switch/3
  Unit Delay/1 -> Lateral Controller Stanley/7
  curvature/1 -> Lateral Controller Stanley/5

== system vehicle_hostmodel_2022b/Controllers/Longitudinal Controllers ==
  Curr Velocity : Inport
  Relative velocity : Inport  Port=2
  Relative distance : Inport  Port=3
  Time gap : Inport  Port=4
  Set velocity : Inport  Port=5
  CurrVel : Inport  Port=6
  Direction : Inport  Port=7
  Adaptive Cruise Control System : mpcadaslib/Adaptive Cruise Control System  EgoModel=tf(1,[0.5,1,0])  InitialEgoVelocity=0  DefaultSpacing=WB+2  MaxVelocity=50  MinAcceleration=-40  amin_ext=off  MaxAcceleration=40  amax_ext=off  Ts=0.1  PredictionHorizon=10  ControllerBehavior=1.0  suboptimal=off  maxiter=10  datatypeopt=double  optmode=off  trackmode=off
  Constant3 : Constant  Value=0
  Longitudinal Controller Stanley : drivingvehiclecontroller/Longitudinal Controller Stanley  Kp=5  Ki=2  SampleTime=0.05  MaxAcceleration=40  MaxDeceleration=40
  Longitudinal acceleration : Outport
  AccelCmd : Outport  Port=2
  DecelCmd : Outport  Port=3
  wires:
  Set velocity/1 -> Longitudinal Controller Stanley/1, Adaptive Cruise Control System/1
  Constant3/1 -> Longitudinal Controller Stanley/4
  Curr Velocity/1 -> Adaptive Cruise Control System/3
  CurrVel/1 -> Longitudinal Controller Stanley/2
  Longitudinal Controller Stanley/1 -> AccelCmd/1
  Longitudinal Controller Stanley/2 -> DecelCmd/1
  Direction/1 -> Longitudinal Controller Stanley/3
  Relative velocity/1 -> Adaptive Cruise Control System/5
  Relative distance/1 -> Adaptive Cruise Control System/4
  Adaptive Cruise Control System/1 -> Longitudinal acceleration/1
  Time gap/1 -> Adaptive Cruise Control System/2

== system vehicle_hostmodel_2022b/Controllers/Subsystem3 ==
  ACCaccel_cmd : Inport
  LCaccel_cmd : Inport  Port=2
  LCdeccel_cmd : Inport  Port=3
  Select : Inport  Port=4
  Merge1 : Merge
  Merge2 : Merge
  Subsystem1 : Subsystem
  Subsystem2 : Subsystem
  Switch Case1 : SwitchCase  CaseConditions={1, 0}  ShowDefaultCase=off
  TorgueCm : Outport
  BrakeCm : Outport  Port=2
  wires:
  LCdeccel_cmd/1 -> Subsystem1/2(decc_cmd)
  Subsystem1/2(brake_cm) -> Merge2/2
  Subsystem1/1(torque_cm) -> Merge1/2
  Subsystem2/2(brake_cm) -> Merge2/1
  Switch Case1/1 -> Subsystem2/Action
  Switch Case1/2 -> Subsystem1/Action
  Subsystem2/1(torque_cm) -> Merge1/1
  LCaccel_cmd/1 -> Subsystem1/1(acc_cmd)
  Merge2/1 -> BrakeCm/1
  ACCaccel_cmd/1 -> Subsystem2/1(acc_cmd)
  Merge1/1 -> TorgueCm/1
  Select/1 -> Switch Case1/1

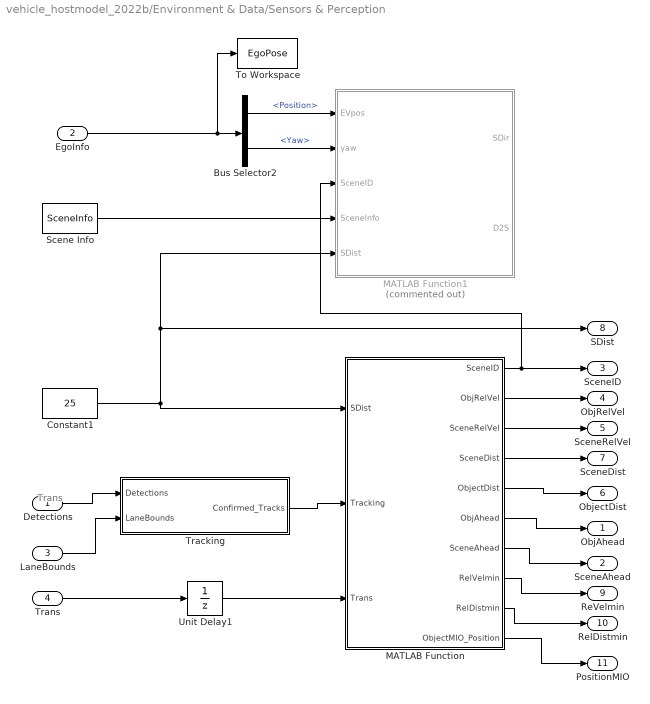
== system vehicle_hostmodel_2022b/Environment & Data/Sensors & Perception ==
  note: Trans
  Detections : Inport
  EgoInfo : Inport  Port=2
  LaneBounds : Inport  Port=3
  Trans : Inport  Port=4
  Bus Selector2 : BusSelector  OutputSignals=Position,Yaw
  Constant1 : Constant  Value=25
  MATLAB Function : MATLAB Function  TreatAsAtomicUnit=on
  MATLAB Function1 : MATLAB Function  Commented=on  TreatAsAtomicUnit=on
  Scene Info : Constant  Value=SceneInfo  VectorParams1D=off
  To Workspace : ToWorkspace  VariableName=EgoPose  SaveFormat=Timeseries  SampleTime=-1
  Tracking : Subsystem
  Unit Delay1 : UnitDelay  SampleTime=0.05  HasFrameUpgradeWarning=on
  ObjAhead : Outport
  SceneAhead : Outport  Port=2
  SceneID : Outport  Port=3
  ObjRelVel : Outport  Port=4
  SceneRelVel : Outport  Port=5
  ObjectDist : Outport  Port=6
  SceneDist : Outport  Port=7
  SDist : Outport  Port=8
  ReVelmin : Outport  Port=9
  RelDistmin : Outport  Port=10
  PositionMIO : Outport  Port=11
  wires:
  MATLAB Function/6(ObjAhead) -> ObjAhead/1
  MATLAB Function/5(ObjectDist) -> ObjectDist/1
  MATLAB Function/7(SceneAhead) -> SceneAhead/1
  MATLAB Function/2(ObjRelVel) -> ObjRelVel/1
  EgoInfo/1 -> To Workspace/1, Bus Selector2/1
  Bus Selector2/1 -> MATLAB Function1/1(EVpos)  "<Position>"
  Detections/1 -> Tracking/1(Detections)
  Scene Info/1 -> MATLAB Function1/4(SceneInfo)
  Bus Selector2/2 -> MATLAB Function1/2(yaw)  "<Yaw>"
  Tracking/1(Confirmed_Tracks) -> MATLAB Function/2(Tracking)
  Constant1/1 -> MATLAB Function1/5(SDist), SDist/1, MATLAB Function/1(SDist)
  MATLAB Function/1(SceneID) -> MATLAB Function1/3(SceneID), SceneID/1
  MATLAB Function/4(SceneDist) -> SceneDist/1
  MATLAB Function/3(SceneRelVel) -> SceneRelVel/1
  MATLAB Function/8(RelVelmin) -> ReVelmin/1
  MATLAB Function/9(RelDistmin) -> RelDistmin/1
  Trans/1 -> Unit Delay1/1
  Unit Delay1/1 -> MATLAB Function/3(Trans)
  LaneBounds/1 -> Tracking/2(LaneBounds)
  MATLAB Function/10(ObjectMIO_Position) -> PositionMIO/1

== system vehicle_hostmodel_2022b/Environment & Data/Subsystem1 ==
  VehFdbk : Inport
  Bus Selector : BusSelector  OutputSignals=InertFrm.Cg.Disp.X,InertFrm.Cg.Disp.Y,InertFrm.Cg.Ang.psi
  Gain1 : Gain  Gain=180/pi
  Mux : Mux  Inputs=3
  Transpose : Math  Operator=transpose  SignedPower=on
  pose : Outport
  wires:
  Mux/1 -> Transpose/1
  VehFdbk/1 -> Bus Selector/1
  Gain1/1 -> Mux/3
  Transpose/1 -> pose/1
  Bus Selector/3 -> Gain1/1  "<psi>"
  Bus Selector/2 -> Mux/2  "<Y>"
  Bus Selector/1 -> Mux/1  "<X>"

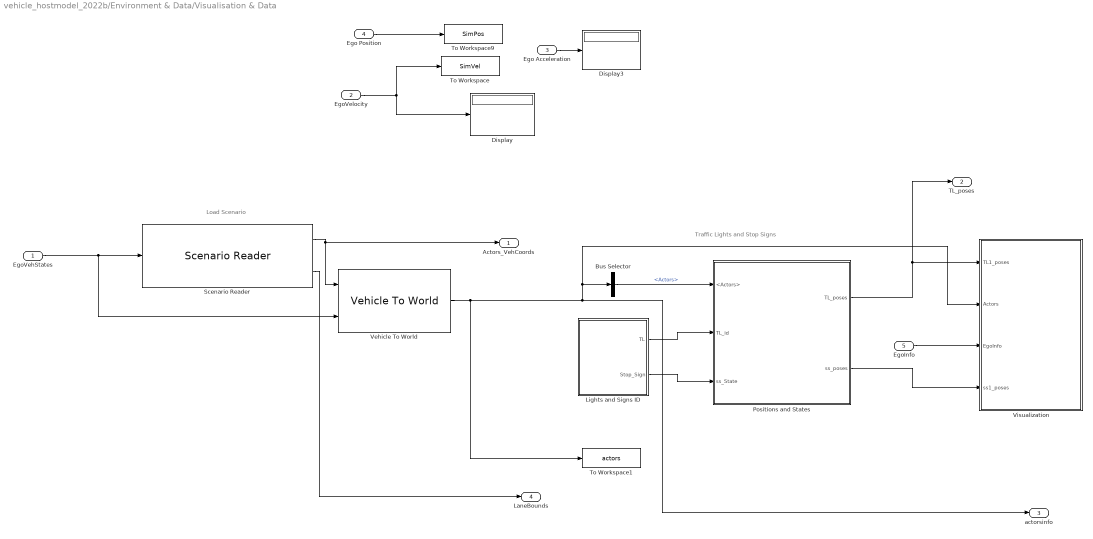
== system vehicle_hostmodel_2022b/Environment & Data/Visualisation & Data ==
  note: Load Scenario
  note: Traffic Lights and Stop Signs
  EgoVehStates : Inport
  EgoVelocity : Inport  Port=2
  Ego Acceleration : Inport  Port=3
  Ego Position : Inport  Port=4
  EgoInfo : Inport  Port=5
  Bus Selector : BusSelector  OutputSignals=Actors
  Display : Display
  Display3 : Display
  Lights and Signs ID : Subsystem
  "Positions and States " : Subsystem
  Scenario Reader : drivingscenarioandsensors/Scenario Reader  ScenarioSource=From file  ScenarioFileName=\\coeit.osu.edu\home\g\giridhar.9\Documents\ADC_Y2\planningControl-Simulation\scenarios\highway_scenario.mat  ScenarioVariableName=scenario  OutputCoordinateSystem=Vehicle coordinates  EgoVehicleSource=Input port  EgoVehicleActorID=1  OrientVehiclesOnRoad=on  OutputEgoVehiclePose=on  OutputEgoVehicleState=off  SampleTime=Ts  LaneBoundaryOutput=All lane boundaries  LaneBoundaryDistance=0:0.5:9.5  LaneBoundaryLocation=Center of lane markings  BusNameSource=Auto  BusName=BusActors  BusNumActorsSource=Scenario  BusNumActors=100  BusName2Source=Auto  BusName2=BusLaneBoundaries  BusNumLaneBoundariesSource=Scenario  BusNumLaneBoundaries=10  BusName3Source=Auto  BusName3=BusEgoActor  BusName4Source=Auto  BusName4=BusEgoState  ShowCoordinateLabels=on  SimulateUsing=Interpreted execution
  To Workspace : ToWorkspace  VariableName=SimVel  SampleTime=-1
      settings: Save2DSignal=2-D array (concatenate along first dimension)
  To Workspace1 : ToWorkspace  VariableName=actors  SaveFormat=Timeseries  SampleTime=-1
  To Workspace9 : ToWorkspace  VariableName=SimPos  SampleTime=-1
      settings: Save2DSignal=2-D array (concatenate along first dimension)
  Vehicle To World : drivingscenarioandsensors/Vehicle To World  BusNameSource=Auto  BusName=BusVehicleToWorldActors  SimulateUsing=Interpreted execution
  Visualization : Subsystem
  Actors_VehCoords : Outport
  TL_poses : Outport  Port=2
  actorsinfo : Outport  Port=3
  LaneBounds : Outport  Port=4
  wires:
  Vehicle To World/1 -> To Workspace1/1, actorsinfo/1, Bus Selector/1, Visualization/2(Actors)
  EgoVelocity/1 -> To Workspace/1, Display/1
  Scenario Reader/1 -> Vehicle To World/1, Actors_VehCoords/1
  "Positions and States "/1(TL_poses) -> TL_poses/1, Visualization/1(TL1_poses)
  Lights and Signs ID/1(TL) -> "Positions and States "/2(TL_id)
  Lights and Signs ID/2(Stop_Sign) -> "Positions and States "/3(ss_State)
  "Positions and States "/2(ss_poses) -> Visualization/4(ss1_poses)
  Ego Acceleration/1 -> Display3/1
  Ego Position/1 -> To Workspace9/1
  EgoInfo/1 -> Visualization/3(EgoInfo)
  EgoVehStates/1 -> Vehicle To World/2, Scenario Reader/1
  Bus Selector/1 -> "Positions and States "/1(<Actors>)  "<Actors>"
  Scenario Reader/2 -> LaneBounds/1

== system vehicle_hostmodel_2022b/Reference Data/Subsystem1 ==
  Input : Inport
  Input1 : Inport  Port=2
  VelFdbk : Inport  Port=3
  Action Port : ActionPort  ActionPortLabel=case [ 1 ]:
  Matrix Concatenate : Concatenate  Mode=Multidimensional array  ConcatenateDimension=2
  Subsystem : Subsystem
  To Workspace : ToWorkspace  VariableName=refPose2  SaveFormat=Timeseries  SampleTime=-1
  RefPos2 : Outport
  RefPose : Outport  Port=2
  DirectionO : Outport  Port=3
  CurvatureO : Outport  Port=4
  wires:
  Matrix Concatenate/1 -> To Workspace/1, RefPos2/1
  Input/1 -> Matrix Concatenate/1
  Input1/1 -> Matrix Concatenate/2
  Subsystem/3(CurvatureO) -> CurvatureO/1
  Subsystem/2(Out2) -> RefPose/1
  Subsystem/4(DirectionO) -> DirectionO/1
  VelFdbk/1 -> Subsystem/1(In1)

== system vehicle_hostmodel_2022b/Reference Data/Subsystem2 ==
  VelFdbk : Inport
  Action Port : ActionPort  ActionPortLabel=case [ 0 ]:
  Subsystem : Subsystem
  RefPose : Outport
  DirectionO : Outport  Port=2
  CurvatureO : Outport  Port=3
  WayPoints : Outport  Port=4
  wires:
  Subsystem/1(Out1) -> WayPoints/1
  Subsystem/4(DirectionO) -> DirectionO/1
  VelFdbk/1 -> Subsystem/1(In1)
  Subsystem/2(Out2) -> RefPose/1
  Subsystem/3(CurvatureO) -> CurvatureO/1

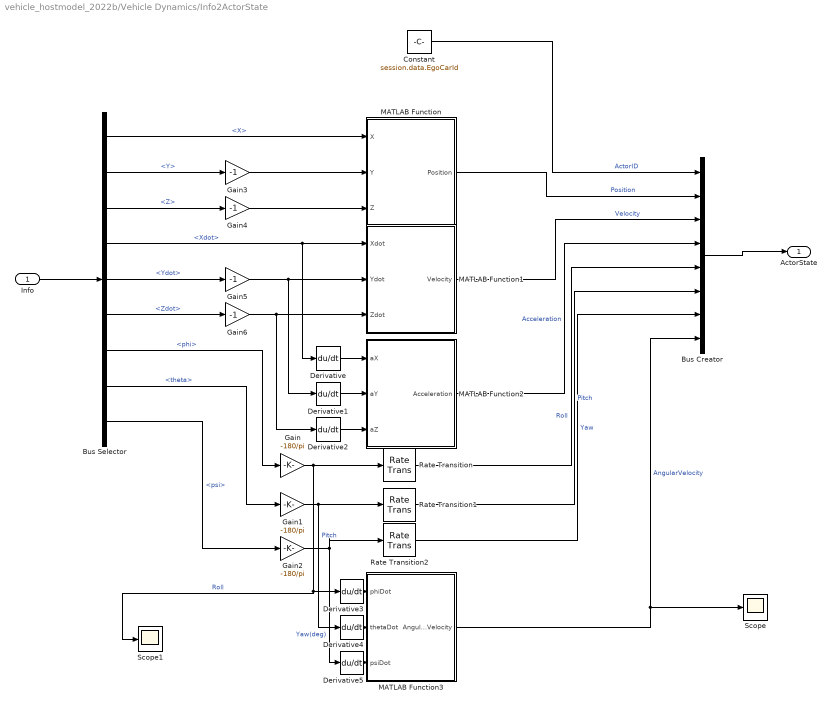
== system vehicle_hostmodel_2022b/Vehicle Dynamics/Info2ActorState ==
  Info : Inport
  Bus Creator : BusCreator  Inputs=ActorID,Position,Velocity,Acceleration,Roll,Pitch,Yaw,AngularVelocity  OutDataTypeStr=Bus: BusActorState  NonVirtualBus=on
  Bus Selector : BusSelector  OutputSignals=InertFrm.Cg.Disp.X,InertFrm.Cg.Disp.Y,InertFrm.Cg.Disp.Z,InertFrm.Cg.Vel.Xdot,InertFrm.Cg.Vel.Ydot,InertFrm.Cg.Vel.Zdot,InertFrm.Cg.Ang.phi,InertFrm.Cg.Ang.theta,InertFrm.Cg.Ang.psi
  Constant : Constant  Value=session.data.EgoCarId  SampleTime=0.05
  Derivative{,1..5} (6 alike) : Derivative
  Gain : Gain  Gain=-180/pi
  Gain1 : Gain  Gain=-180/pi
  Gain2 : Gain  Gain=-180/pi
  Gain{3..6} (4 alike) : Gain  Gain=-1
  MATLAB Function : MATLAB Function  TreatAsAtomicUnit=on  SystemSampleTime=0.05
  MATLAB Function1 : MATLAB Function  TreatAsAtomicUnit=on  SystemSampleTime=0.05
  MATLAB Function2 : MATLAB Function  TreatAsAtomicUnit=on  SystemSampleTime=0.05
  MATLAB Function3 : MATLAB Function  TreatAsAtomicUnit=on  SystemSampleTime=0.05
  Rate Transition : RateTransition  OutPortSampleTime=0.05
  Rate Transition1 : RateTransition  OutPortSampleTime=0.05
  Rate Transition2 : RateTransition  OutPortSampleTime=0.05
  Scope : Scope
  Scope1 : Scope
  ActorState : Outport
  wires:
  Gain/1 -> Scope1/1, Derivative3/1, Rate Transition/1  "Roll"
  Derivative4/1 -> MATLAB Function3/2(thetaDot)
  Bus Selector/2 -> Gain3/1  "<Y>"
  Bus Selector/4 -> Derivative/1, MATLAB Function1/1(Xdot)  "<Xdot>"
  MATLAB Function1/1(Velocity) -> Bus Creator/3  "Velocity"
  MATLAB Function/1(Position) -> Bus Creator/2  "Position"
  Derivative1/1 -> MATLAB Function2/2(aY)
  Bus Selector/5 -> Gain5/1  "<Ydot>"
  Bus Selector/1 -> MATLAB Function/1(X)  "<X>"
  Bus Selector/9 -> Gain2/1  "<psi>"
  Gain2/1 -> Rate Transition2/1, Derivative5/1  "Yaw(deg)"
  Derivative5/1 -> MATLAB Function3/3(psiDot)
  Bus Selector/7 -> Gain/1  "<phi>"
  MATLAB Function2/1(Acceleration) -> Bus Creator/4  "Acceleration"
  Derivative3/1 -> MATLAB Function3/1(phiDot)
  Gain1/1 -> Derivative4/1, Rate Transition1/1  "Pitch"
  Bus Selector/6 -> Gain6/1  "<Zdot>"
  Bus Selector/8 -> Gain1/1  "<theta>"
  MATLAB Function3/1(AngularVelocity) -> Bus Creator/8, Scope/1  "AngularVelocity"
  Bus Selector/3 -> Gain4/1  "<Z>"
  Derivative2/1 -> MATLAB Function2/3(aZ)
  Derivative/1 -> MATLAB Function2/1(aX)
  Info/1 -> Bus Selector/1
  Constant/1 -> Bus Creator/1  "ActorID"
  Bus Creator/1 -> ActorState/1
  Rate Transition/1 -> Bus Creator/5  "Roll"
  Rate Transition1/1 -> Bus Creator/6  "Pitch"
  Rate Transition2/1 -> Bus Creator/7  "Yaw"
  Gain3/1 -> MATLAB Function/2(Y)
  Gain4/1 -> MATLAB Function/3(Z)
  Gain5/1 -> Derivative1/1, MATLAB Function1/2(Ydot)
  Gain6/1 -> Derivative2/1, MATLAB Function1/3(Zdot)

== system vehicle_hostmodel_2022b/Vehicle Dynamics/Subsystem ==
  Gain : Gain  Gain=MAX_TORQUE*0.1
  Gain1 : Gain  Gain=MIN_BRAKE*0.06
  Gain2 : Gain  Gain=MAX_STEER/4.5
  Signal Builder : Subsystem  Tag=STV Subsys  LoadFcn=sigbuilder_block('load');  StartFcn=sigbuilder_block('start');  StopFcn=sigbuilder_block('stop');  ClipboardFcn=sigbuilder_block('clipboard');  mask(Sigbuilder block){tuvar=[0:10]}
      mask help: Simulink:masks:SigbuilderBlock_MD
      mask init:
      | if ~strcmp(get_param(bdroot(gcbh),'SimulationStatus'),'stopped') tuvar = sigbuilder_block('maskInit'); end
      settings: CopyFcn=sigbuilder_block('copy');  DeleteFcn=sigbuilder_block('delete');  ModelCloseFcn=sigbuilder_block('modelClose');  PreSaveFcn=sigbuilder_block('preSave');  PauseFcn=sigbuilder_block('pause');  ContinueFcn=sigbuilder_block('continue');  NameChangeFcn=sigbuilder_block('namechange');  OpenFcn=sigbuilder_block('open',[0 30 960 455.5 ]);  CloseFcn=sigbuilder_block('close');
      mask Display: plot(0, 0, 100, 100,[2, 2, 32, 32, 2], [68, 8, 8, 68, 68],[32, 2], [38, 38], [32, 19, 2],[53, 60, 44], [32, 17, 17, 2],[16, 16, 31, 31]);txt = getActiveGroup(gcbh);text(2, 100, txt,'verticalAlignment', 'top');
  torque_cmd (Nm) : Outport
  brake_cmd (Nm) : Outport  Port=2
  steer_cmd (deg) : Outport  Port=3
  wires:
  Gain2/1 -> steer_cmd (deg)/1  "steer_cmd (deg)"
  Signal Builder/1(Normalized Torque) -> Gain/1
  Signal Builder/2(Normalized Brake) -> Gain1/1
  Signal Builder/3(Normalized Steer) -> Gain2/1  "steer_cmd (deg)"
  Gain1/1 -> brake_cmd (Nm)/1  "brake_cmd (Nm)"
  Gain/1 -> torque_cmd (Nm)/1  "torque_cmd (Nm)"

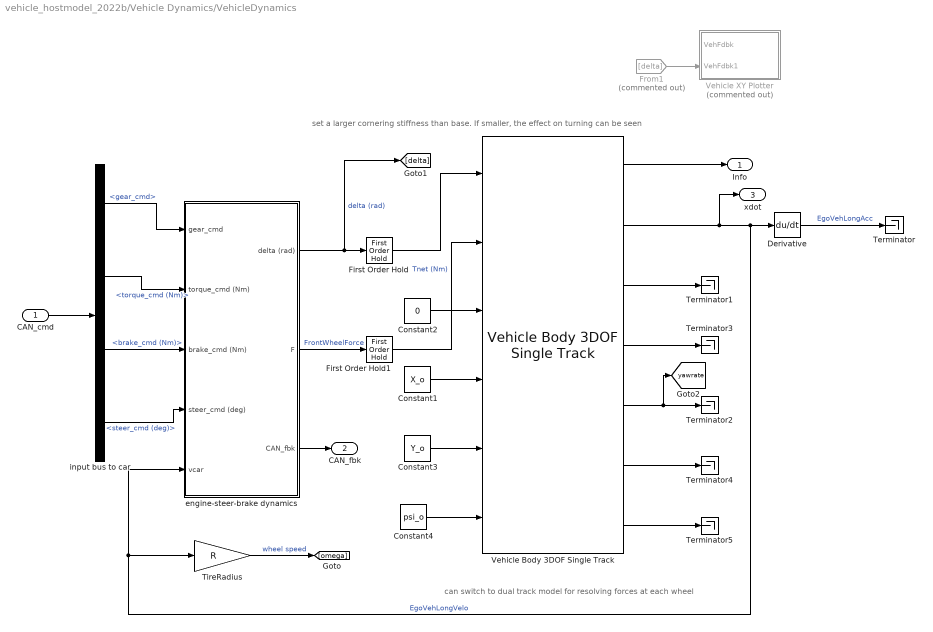
== system vehicle_hostmodel_2022b/Vehicle Dynamics/VehicleDynamics ==
  note: set a larger cornering stiffness than base. If smaller, the effect on turning can be seen
  note: can switch to dual track model for resolving forces at each wheel
  CAN_cmd : Inport
  Constant1 : Constant  Value=X_o
  Constant2 : Constant  Value=0
  Constant3 : Constant  Value=Y_o
  Constant4 : Constant  Value=psi_o
  Derivative : Derivative
  First Order Hold : FirstOrderHold  ErrorTolerance=inf
  First Order Hold1 : FirstOrderHold  ErrorTolerance=inf
  From1 : From  Commented=on  GotoTag=delta
  Terminator{,1..5} (6 alike) : Terminator
  TireRadius : Gain  Gain=R
  Vehicle Body 3DOF Single Track : autolibshared/Vehicle Body 3DOF Single Track  trackMode=Single (bicycle)  inputMode=External longitudinal forces  frontSteerMode=on  rearSteerMode=off  windMode=off  muMode=off  extFMode=off  extMMode=off  htchFMode=off  htchMMode=off  extXo=on  extpsio=on  extxdoto=off  extro=off  extYo=on  extTamb=off  extydoto=off  aMode=2  NF=2  NR=2  m=MCAR  a=LF  b=LR  h=0.35  dh=1  hh=0.2  X_o=InitPosition(1)  xdot_o=InitSpeed  CalphaMode=off  sigmaMode=on  d=0  hl=0  w=[1.4,1.4]  Cy_f=12e3*100  Cy_r=11e3*100  sigma_f=.1  sigma_r=.1  alpha_f_brk=[-.1 .1]  Cy_f_data=[-9e3 9e3]  alpha_r_brk=[-.1 .1]  Cy_r_data=[-9e3 9e3]  Y_o=-InitPosition(2)  ydot_o=0  Izz=2050  psi_o=-InitYaw/180*pi  r_o=0  Af=2  Cd=.3  Cl=.1  Cpm=.1  beta_w=[0:0.01:0.3]  Cs=[0:0.03:0.9]  Cym=[0:0.01:0.3]  Pabs=101325  Tair=273  g=9.81  mu=1  xdot_tol=.01  Fznom=5000  Fxtire_sat=7e4  Fytire_sat=7e4  longOff=0  latOff=0  vertOff=0  wrapAng=off
  Vehicle XY Plotter : Subsystem  Commented=on  mask(Vehicle XY Plotter){a=LF, b=LR, w=TrackWidth, bufferSize=1024, pltDT=.1}
      mask prompts: a "Distance to front axle from CG, a [m]:"; b "Distance to rear axle from CG, b [m]:"; w "Track width, w [m]:"; bufferSize "Path buffer sampe size, bufferSize []:"; pltDT "Plot update rate, pltDT [s]:"
      mask help: This block will display a MATLAB figure which indicates the vehicle path, current position and heading velocity.
      mask TypeOptions a: Vehicle XY Plotter/a
      mask TypeOptions b: Vehicle XY Plotter/b
      mask TypeOptions w: Vehicle XY Plotter/w
      mask TypeOptions bufferSize: Vehicle XY Plotter/bufferSize
  engine-steer-brake dynamics : Subsystem
  input bus to car : BusSelector  OutputSignals=gear_cmd,torque_cmd (Nm),brake_cmd (Nm),steer_cmd (deg)
  Info : Outport
  CAN_fbk : Outport  Port=2  VectorParamsAs1DForOutWhenUnconnected=off
  xdot : Outport  Port=3
  tag scope: yawrate=global
  wires:
  TireRadius/1 -> [omega]  "wheel speed"
  Vehicle Body 3DOF Single Track/1 -> Info/1
  From1/1 -> Vehicle XY Plotter/2(VehFdbk1)
  input bus to car/1 -> engine-steer-brake dynamics/1(gear_cmd)  "<gear_cmd>"
  input bus to car/3 -> engine-steer-brake dynamics/3(brake_cmd (Nm))  "<brake_cmd (Nm)>"
  engine-steer-brake dynamics/1(delta (rad)) -> [delta], First Order Hold/1  "delta (rad)"
  input bus to car/2 -> engine-steer-brake dynamics/2(torque_cmd (Nm))  "<torque_cmd (Nm)>"
  input bus to car/4 -> engine-steer-brake dynamics/4(steer_cmd (deg))  "<steer_cmd (deg)>"
  engine-steer-brake dynamics/3(CAN_fbk) -> CAN_fbk/1
  CAN_cmd/1 -> input bus to car/1
  Constant2/1 -> Vehicle Body 3DOF Single Track/3
  engine-steer-brake dynamics/2(F) -> First Order Hold1/1  "FrontWheelForce"
  First Order Hold/1 -> Vehicle Body 3DOF Single Track/1
  Vehicle Body 3DOF Single Track/2 -> xdot/1, engine-steer-brake dynamics/5(vcar), TireRadius/1, Derivative/1  "EgoVehLongVelo"
  Vehicle Body 3DOF Single Track/3 -> Terminator1/1
  Vehicle Body 3DOF Single Track/4 -> Terminator3/1
  Vehicle Body 3DOF Single Track/5 -> [yawrate], Terminator2/1
  Vehicle Body 3DOF Single Track/6 -> Terminator4/1
  Vehicle Body 3DOF Single Track/7 -> Terminator5/1
  Derivative/1 -> Terminator/1  "EgoVehLongAcc"
  First Order Hold1/1 -> Vehicle Body 3DOF Single Track/2  "Tnet (Nm)"
  Constant1/1 -> Vehicle Body 3DOF Single Track/4
  Constant3/1 -> Vehicle Body 3DOF Single Track/5
  Constant4/1 -> Vehicle Body 3DOF Single Track/6
